simulink model "BDot"  (R2015b)
settings: Solver=ode45  StartTime=0.0  StopTime=tprop  RelTol=1e-3
values from neighbouring files (symbols this model uses):
  J = [(1/12)*m*h^2 0 0 ; 0 (1/12)*m*h^2 0; 0 0 .5*m*r^2]    [SetUp.m]
  Jinv = inv(J)    [SetUp.m]
  kd = J*2*zeta*nf    [SetUp.m]
  mu = 398600    [COES2rvd.m]    (also in SetUp.m; test.m)
  rvect = invconvmat*rvectx    [COES2rvd.m]    (also in test.m = rvect')
  TcON = 1    [SetUp.m]
  Tcy = [0 kd(2,2)*(.5*mw*rw^2)*capOmega 0]    [SetUp.m]
  TcyON = 0    [SetUp.m]
  vvect = invconvmat*vvectx    [COES2rvd.m]    (also in test.m = vvect')
  wbn0 = DCM*w    [SetUp.m]
undefined symbols (not defined in the file or in its folder): IAU
libraries: aerolibtransform2 x1, aerolibgravity2 x1
settings Model: Creator=Trent  LastModifiedBy=morganyost
settings DataIOCC: SaveFormat=Array
settings HardwareCC: ProdBitPerPointer=32  ProdLargestAtomicFloat=None  ProdIntDivRoundTo=Undefined  ProdEndianess=Unspecified  ProdWordSize=32  ProdHWDeviceType=32-bit Generic
settings GRTTargetCC: GeneratePreprocessorConditionals=Disable all
settings ConfigComp: CovModelRefEnable=Off

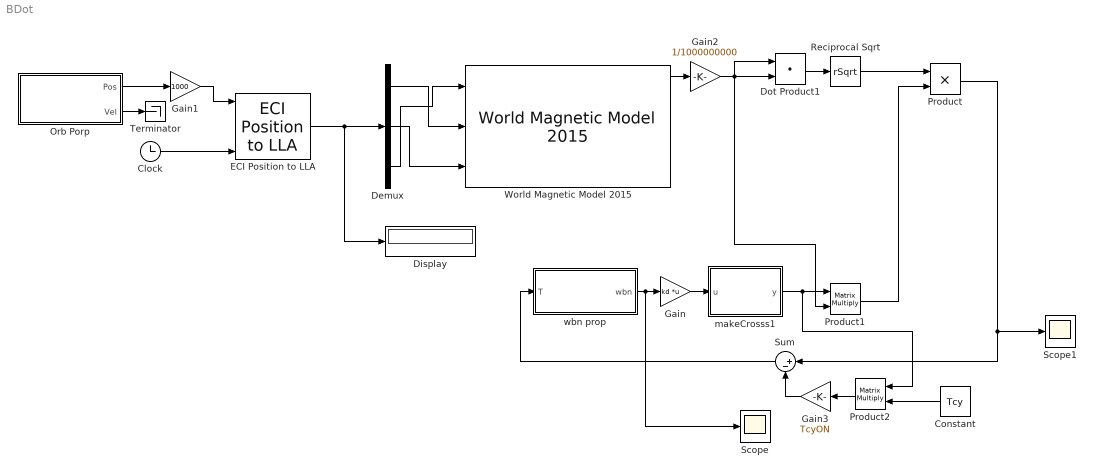
== system BDot ==
  Clock : Clock
  Constant : Constant  Value=Tcy
  Demux : Demux  Outputs=3
  Display : Display
  Dot Product1 : DotProduct  InputSameDT=on  OutDataTypeStr=Inherit: Inherit via internal rule
  ECI Position to LLA : aerolibtransform2/ECI Position to LLA  red=IAU-2000/2006  year=2015  month=December  day=2  hour=0  min=0  sec=0  deltaT=Sec  errorflag=Error  extraparamflag=on  eunits=Metric (MKS)  earthmodel=WGS84  flat=1/298.257223563  eqradius=6378137
      settings: AttributesFormatString=%<red>
  Gain : Gain  Gain=kd  Multiplication=Matrix(K*u) (u vector)
  Gain1 : Gain  Gain=1000
  Gain2 : Gain  Gain=1/1000000000
  Gain3 : Gain  Gain=TcyON
  Orb Porp : Subsystem
  Product : Product
  Product1 : Product  Multiplication=Matrix(*)
  Product2 : Product  Multiplication=Matrix(*)
  Reciprocal Sqrt : Sqrt  Operator=rSqrt  SaturateOnIntegerOverflow=on
  Scope : Scope
  Scope1 : Scope
  Sum : Sum  Inputs=|+-
  Terminator : Terminator
  World Magnetic Model 2015 : aerolibgravity2/World Magnetic Model 2015  RequirementInfo="{}  %GIDa_c707c699_7679_46e8_b9d9_c8e087eee6a8"  units=Metric (MKS)  time_in=off  month=December  day=2  year=2015  action=Error  h_out=on  dec_out=on  inc_out=on  ti_out=on
  makeCrosss1 : MATLAB Function  TreatAsAtomicUnit=on
  wbn prop : Subsystem
  wires:
  ECI Position to LLA/1 -> Display/1, Demux/1
  Clock/1 -> ECI Position to LLA/6
  World Magnetic Model 2015/1 -> Gain2/1
  Dot Product1/1 -> Reciprocal Sqrt/1
  Reciprocal Sqrt/1 -> Product/1
  wbn prop/1(wbn) -> Scope/1, Gain/1
  Gain/1 -> makeCrosss1/1(u)
  makeCrosss1/1(y) -> Product2/1, Product1/1
  Product1/1 -> Product/2
  Product/1 -> Sum/1, Scope1/1
  Orb Porp/2(Vel) -> Terminator/1
  Demux/1 -> World Magnetic Model 2015/2
  Demux/2 -> World Magnetic Model 2015/3
  Demux/3 -> World Magnetic Model 2015/1
  Orb Porp/1(Pos) -> Gain1/1
  Gain1/1 -> ECI Position to LLA/1
  Gain2/1 -> Dot Product1/1, Dot Product1/2, Product1/2
  Constant/1 -> Product2/2
  Product2/1 -> Gain3/1
  Sum/1 -> wbn prop/1(T)
  Gain3/1 -> Sum/2

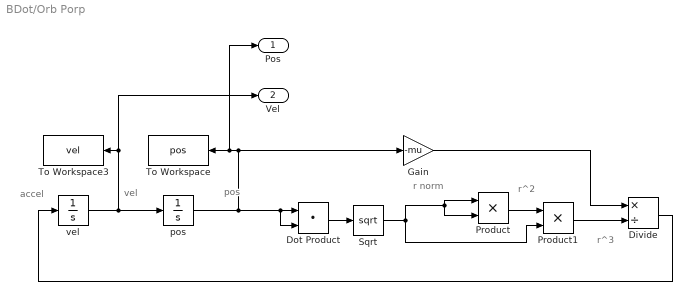
== system BDot/Orb Porp ==
  note: r^3
  note: r^2
  note: r norm
  note: pos
  note: vel
  note: accel
  Divide : Product  Inputs=*/
  Dot Product : DotProduct  InputSameDT=on  OutDataTypeStr=Inherit: Inherit via internal rule
  Gain : Gain  Gain=-mu
  Product : Product
  Product1 : Product
  Sqrt : Sqrt  SaturateOnIntegerOverflow=on
  To Workspace : ToWorkspace  VariableName=pos  SaveFormat=Timeseries  SampleTime=-1
  To Workspace3 : ToWorkspace  VariableName=vel  SaveFormat=Timeseries  SampleTime=-1
  pos : Integrator  InitialCondition=rvect
  vel : Integrator  InitialCondition=vvect
  Pos : Outport
  Vel : Outport  Port=2
  wires:
  vel/1 -> Vel/1, To Workspace3/1, pos/1
  pos/1 -> Gain/1, Pos/1, To Workspace/1, Dot Product/2, Dot Product/1
  Sqrt/1 -> Product/2, Product/1, Product1/2
  Product/1 -> Product1/1
  Product1/1 -> Divide/2
  Gain/1 -> Divide/1
  Divide/1 -> vel/1
  Dot Product/1 -> Sqrt/1

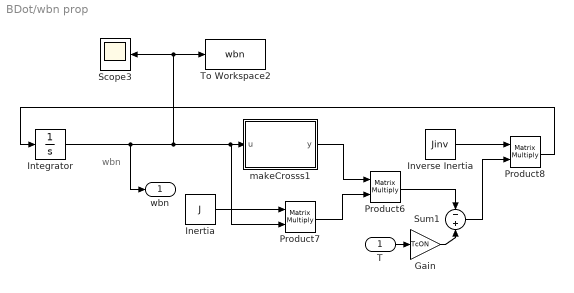
== system BDot/wbn prop ==
  note: wbn
  T : Inport
  Gain : Gain  Gain=TcON
  Inertia : Constant  Value=J
  Integrator : Integrator  InitialCondition=wbn0
  Inverse Inertia : Constant  Value=Jinv
  Product6 : Product  Multiplication=Matrix(*)
  Product7 : Product  Multiplication=Matrix(*)
  Product8 : Product  Multiplication=Matrix(*)
  Scope3 : Scope
  Sum1 : Sum  Inputs=-+
  To Workspace2 : ToWorkspace  VariableName=wbn  SaveFormat=Timeseries  SampleTime=-1
  makeCrosss1 : MATLAB Function  TreatAsAtomicUnit=on
  wbn : Outport
  wires:
  makeCrosss1/1(y) -> Product6/1
  Inertia/1 -> Product7/1
  Product7/1 -> Product6/2
  Inverse Inertia/1 -> Product8/1
  Product8/1 -> Integrator/1
  Product6/1 -> Sum1/1
  Sum1/1 -> Product8/2
  Integrator/1 -> wbn/1, Product7/2, makeCrosss1/1(u), Scope3/1, To Workspace2/1
  T/1 -> Gain/1
  Gain/1 -> Sum1/2

== matlab function BDot/makeCrosss1 ==
  data: u input; y output
function y = fcn(u)
%#codegen
Ex = u(1);
Ey = u(2);
Ez = u(3);

y = [0 -Ez Ey; Ez 0 -Ex; -Ey Ex 0];

== matlab function BDot/wbn prop/makeCrosss1 ==
  data: u input; y output
function y = fcn(u)
%#codegen
Ex = u(1);
Ey = u(2);
Ez = u(3);

y = [0 -Ez Ey; Ez 0 -Ex; -Ey Ex 0];
